simulink model "LaneChangeController"  (R2025b)
settings: Solver=FixedStepAuto  StartTime=0.0  StopTime=10.0  RelTol=1e-3
undefined symbols (not defined in the file): egoInitialPose, predictionHorizon, Ts
libraries: mpcadaslib x1
settings Model: Creator=The MathWorks, Inc.  LastModifiedBy=The MathWorks, Inc.
settings SolverCC: AlgebraicLoopSolver=TrustRegion  MaxZcPerStep=1.0
settings OptimizationCC: DefaultParameterBehavior=Inlined  EnhancedBackFolding=on  PassReuseOutputArgsAs=Individual arguments  ZeroExternalMemoryAtStartup=off  ZeroInternalMemoryAtStartup=off  OptimizeBlockOrder=speed  DifferentSizesBufferReuse=on  OptimizationCustomize=off  EfficientTunableParamExpr=on
settings DebuggingCC: ParameterTunabilityLossMsg=error  UnconnectedInputMsg=warning  UnconnectedOutputMsg=warning  UnconnectedLineMsg=warning  SubsystemReferenceDiagnosticForUnitTest=warning
settings HardwareCC: ProdLongLongMode=on
settings ModelReferenceCC: EnableRefExpFcnMdlSchedulingChecks=on
settings SFSimCC: MATLABDynamicMemAlloc=off
settings RTWCC: SystemTargetFile=ert.tlc  TemplateMakefile=ert_default_tmf  PortableWordSizes=on  TargetLang=C++  GPUComputeCapability=3.5  DLArmComputeVersion=19.05  Description=Embedded Coder
settings CodeAppCC: ForceParamTrailComments=on  IgnoreCustomStorageClasses=off  MaxIdLength=256.0  OperatorAnnotations=on  SimulinkDataObjDesc=on  SFDataObjDesc=on  InsertBlockDesc=on
settings ERTTargetCC: RootIOFormat=Structure reference  ERTCustomFileTemplate=example_file_process.tlc  DynamicArrayContainerType=coder::array  TargetLangStandard=C++03 (ISO)  GenerateSampleERTMain=on  CodeInterfacePackaging=C++ class  SubcomponentCodeInterfacePackaging=C++ class

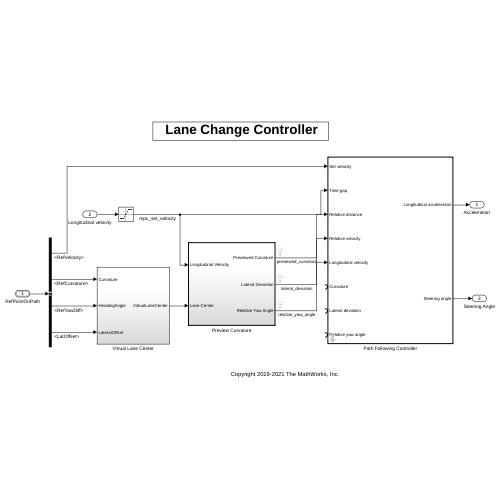
[thumbnail: Simulink's stored preview of the top-level diagram]
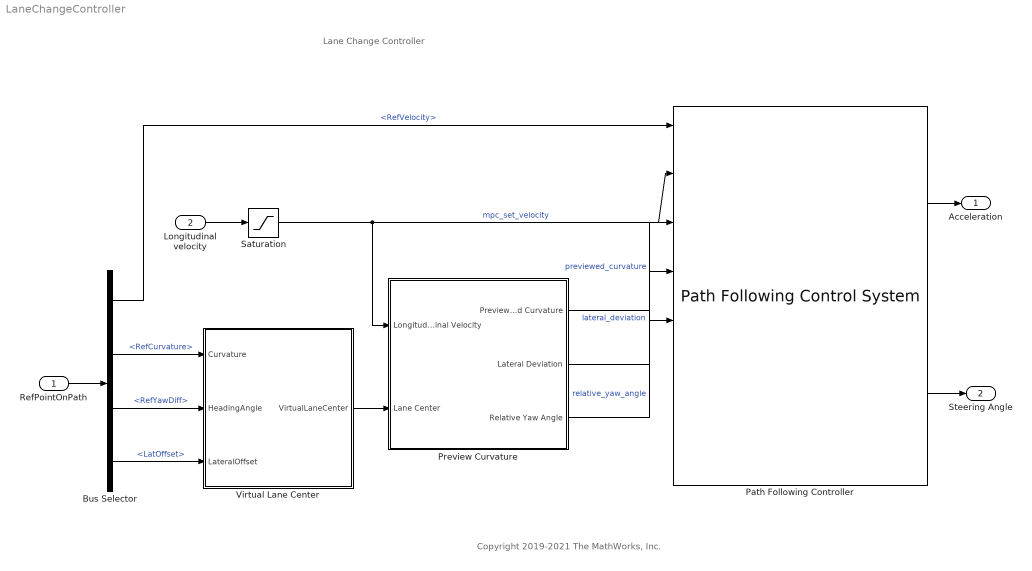
== system LaneChangeController ==
  note: Lane Change Controller
  note: Copyright 2019-2021 The MathWorks, Inc.
  RefPointOnPath : Inport  OutDataTypeStr=Bus: BusRefPointOnPath  BusOutputAsStruct=on
  Longitudinal velocity : Inport  Port=2
  Bus Selector : BusSelector  OutputSignals=RefVelocity,RefCurvature,RefYawDiff,LatOffset
  Path Following Controller : mpcadaslib/Path Following Control System  VariantControl=Variant2  ModelType=Use vehicle parameters  VehicleMass=m  VehicleYawInertia=Iz  LengthToFront=lf  LengthToRear=lr  FrontTireStiffness=Cf  RearTireStiffness=Cr  AccelTimeConstant=tau  EgoModelMatrixA=[-2,zeros(1,3);1,zeros(1,3);zeros(1,2),-4.4021,-12.4603;zeros(1,2),1.3913,-5.1868]  EgoModelMatrixB=[2,zeros(1,3);zeros(1,2),24.1270,15.8609]'  EgoModelMatrixC=[zeros(3,1),eye(3)]  InitialLongVel=hypot(egoInitialPose .Velocity(1), egoInitialPose.Velocity(2));  TransportLag=Ts  spaceCtrl=off  DefaultSpacing=defaultSpacing  MinSteering=minSteer  umin_ext=off  MaxSteering=maxSteer  umax_ext=off  MinAcceleration=min_ac  amin_ext=off  MaxAcceleration=max_ac  amax_ext=off  Ts=Ts  PredictionHorizon=120/Ts*0.1  ControlHorizon=2  LongWeight=0.5  LateralWeight=1  AccelRateWeight=0.1  SteerRateWeight=0.1  suboptimal=off  maxiter=10  datatypeopt=double  optmode=off  trackmode=off
  Preview Curvature : Subsystem  TreatAsAtomicUnit=on
  Saturation : Saturate  UpperLimit=inf  LowerLimit=0.0001
  Virtual Lane Center : Subsystem
  Acceleration : Outport  VectorParamsAs1DForOutWhenUnconnected=off
  Steering Angle : Outport  Port=2  VectorParamsAs1DForOutWhenUnconnected=off
  wires:
  Preview Curvature/1(Previewed Curvature) -> Path Following Controller/3  "previewed_curvature"
  Preview Curvature/2(Lateral Deviation) -> Path Following Controller/4  "lateral_deviation"
  Bus Selector/3 -> Virtual Lane Center/2(HeadingAngle)  "<RefYawDiff>"
  Saturation/1 -> Path Following Controller/2, Preview Curvature/1(Longitudinal Velocity)  "mpc_set_velocity"
  Longitudinal velocity/1 -> Saturation/1
  RefPointOnPath/1 -> Bus Selector/1
  Bus Selector/1 -> Path Following Controller/1  "<RefVelocity>"
  Preview Curvature/3(Relative Yaw Angle) -> Path Following Controller/5  "relative_yaw_angle"
  Bus Selector/4 -> Virtual Lane Center/3(LateralOffset)  "<LatOffset>"
  Path Following Controller/1 -> Acceleration/1
  Bus Selector/2 -> Virtual Lane Center/1(Curvature)  "<RefCurvature>"
  Virtual Lane Center/1(VirtualLaneCenter) -> Preview Curvature/2(Lane Center)
  Path Following Controller/2 -> Steering Angle/1

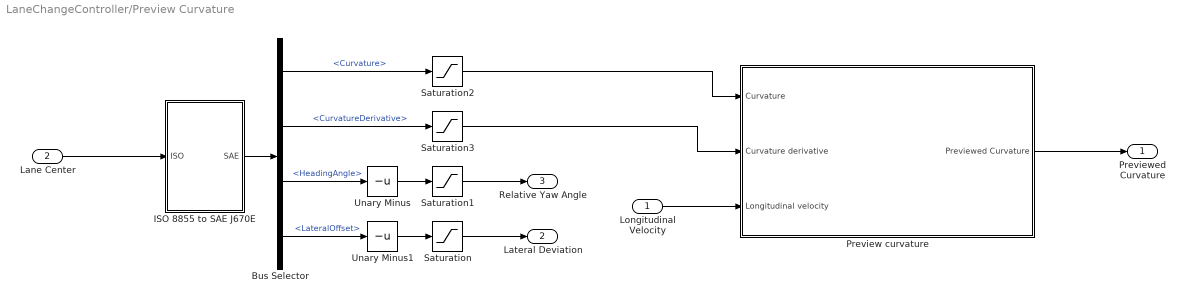
== system LaneChangeController/Preview Curvature ==
  Longitudinal Velocity : Inport
  Lane Center : Inport  Port=2
  Bus Selector : BusSelector  OutputSignals=Curvature,CurvatureDerivative,HeadingAngle,LateralOffset
  ISO 8855 to SAE J670E : Subsystem
  Preview curvature : Subsystem
  Saturation : Saturate
  Saturation1 : Saturate  UpperLimit=0.8  LowerLimit=-0.8
  Saturation2 : Saturate  UpperLimit=0.15  LowerLimit=-0.15
  Saturation3 : Saturate  UpperLimit=0.06  LowerLimit=-0.06
  Unary Minus : UnaryMinus
  Unary Minus1 : UnaryMinus
  Previewed Curvature : Outport  VectorParamsAs1DForOutWhenUnconnected=off
  Lateral Deviation : Outport  Port=2  VectorParamsAs1DForOutWhenUnconnected=off
  Relative Yaw Angle : Outport  Port=3  VectorParamsAs1DForOutWhenUnconnected=off
  wires:
  Bus Selector/4 -> Unary Minus1/1  "<LateralOffset>"
  ISO 8855 to SAE J670E/1(SAE) -> Bus Selector/1
  Unary Minus1/1 -> Saturation/1
  Saturation3/1 -> Preview curvature/2(Curvature derivative)
  Bus Selector/1 -> Saturation2/1  "<Curvature>"
  Unary Minus/1 -> Saturation1/1
  Lane Center/1 -> ISO 8855 to SAE J670E/1(ISO)
  Saturation1/1 -> Relative Yaw Angle/1
  Longitudinal Velocity/1 -> Preview curvature/3(Longitudinal velocity)
  Saturation/1 -> Lateral Deviation/1
  Bus Selector/3 -> Unary Minus/1  "<HeadingAngle>"
  Saturation2/1 -> Preview curvature/1(Curvature)
  Bus Selector/2 -> Saturation3/1  "<CurvatureDerivative>"
  Preview curvature/1(Previewed Curvature) -> Previewed Curvature/1

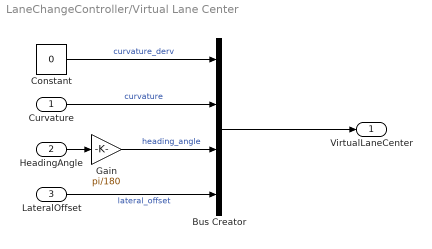
== system LaneChangeController/Virtual Lane Center ==
  Curvature : Inport
  HeadingAngle : Inport  Port=2
  LateralOffset : Inport  Port=3
  Bus Creator : BusCreator  Inputs=4
  Constant : Constant  Value=0
  Gain : Gain  Gain=pi/180
  VirtualLaneCenter : Outport  VectorParamsAs1DForOutWhenUnconnected=off
  wires:
  Bus Creator/1 -> VirtualLaneCenter/1
  Gain/1 -> Bus Creator/3  "heading_angle"
  LateralOffset/1 -> Bus Creator/4  "lateral_offset"
  HeadingAngle/1 -> Gain/1
  Curvature/1 -> Bus Creator/2  "curvature"
  Constant/1 -> Bus Creator/1  "curvature_derv"

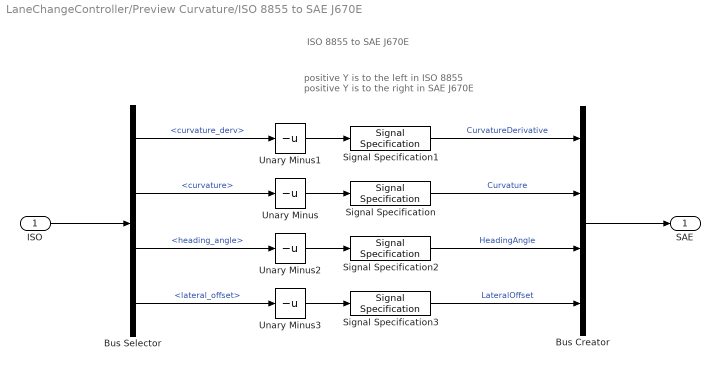
== system LaneChangeController/Preview Curvature/ISO 8855 to SAE J670E ==
  note: positive Y is to the left in ISO 8855
      | positive Y is to the right in SAE J670E
  note: ISO 8855 to SAE J670E
  ISO : Inport
  Bus Creator : BusCreator  Inputs=4
  Bus Selector : BusSelector  OutputSignals=curvature_derv,curvature,heading_angle,lateral_offset
  Signal Specification : SignalSpecification  Unit=1/m
  Signal Specification1 : SignalSpecification  Unit=1/m^2
  Signal Specification2 : SignalSpecification  Unit=rad
  Signal Specification3 : SignalSpecification  Unit=m
  Unary Minus{,1..3} (4 alike) : UnaryMinus
  SAE : Outport  VectorParamsAs1DForOutWhenUnconnected=off
  wires:
  ISO/1 -> Bus Selector/1
  Bus Selector/2 -> Unary Minus/1  "<curvature>"
  Bus Selector/1 -> Unary Minus1/1  "<curvature_derv>"
  Bus Selector/3 -> Unary Minus2/1  "<heading_angle>"
  Bus Selector/4 -> Unary Minus3/1  "<lateral_offset>"
  Bus Creator/1 -> SAE/1
  Signal Specification/1 -> Bus Creator/2  "Curvature"
  Unary Minus1/1 -> Signal Specification1/1
  Unary Minus2/1 -> Signal Specification2/1
  Unary Minus3/1 -> Signal Specification3/1
  Unary Minus/1 -> Signal Specification/1
  Signal Specification1/1 -> Bus Creator/1  "CurvatureDerivative"
  Signal Specification2/1 -> Bus Creator/3  "HeadingAngle"
  Signal Specification3/1 -> Bus Creator/4  "LateralOffset"

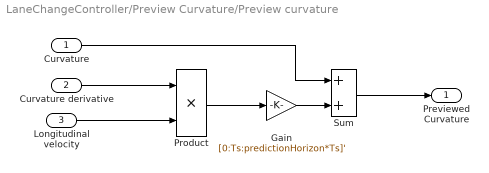
== system LaneChangeController/Preview Curvature/Preview curvature ==
  Curvature : Inport
  Curvature derivative : Inport  Port=2
  Longitudinal velocity : Inport  Port=3
  Gain : Gain  Gain=[0:Ts:predictionHorizon*Ts]'
  Product : Product
  Sum : Sum
  Previewed Curvature : Outport  VectorParamsAs1DForOutWhenUnconnected=off
  wires:
  Sum/1 -> Previewed Curvature/1
  Curvature/1 -> Sum/1
  Gain/1 -> Sum/2
  Product/1 -> Gain/1
  Longitudinal velocity/1 -> Product/2
  Curvature derivative/1 -> Product/1
